simulink model "noizeGen"  (R2016b)
settings: Solver=VariableStepAuto  StartTime=0.0  StopTime=270  RelTol=1e-3
values from neighbouring files (symbols this model uses):
  noisePower = db2pow(-66)    [kalmanData.m]
  peak0amp = 0.0043080+0.0005    (= 0.004808)    [kalmanData.m]
  peak0fq = 0.003701*2*pi    (= 0.0232540688219)    [kalmanData.m]
  peak1amp = 0.0087010+0.0002    (= 0.008901)    [kalmanData.m]
  peak1fq = 0.9919*2*pi    (= 6.23229150619)    [kalmanData.m]
  peak2amp = 0.0023260+0.001    (= 0.003326)    [kalmanData.m]
  peak2fq = 2.979*2*pi    (= 18.7176090301)    [kalmanData.m]
  peak3amp = 0.0015270+0.00027    (= 0.001797)    [kalmanData.m]
  peak3fq = 4.978*2*pi    (= 31.2776964591)    [kalmanData.m]
  peak4amp = 0.0010100+0.0002    (= 0.00121)    [kalmanData.m]
  peak4fq = 6.973*2*pi    (= 43.812651147)    [kalmanData.m]
  peak5amp = 0.0009673+0.00023    (= 0.0011973)    [kalmanData.m]
  peak5fq = 8.96*2*pi    (= 56.2973403523)    [kalmanData.m]
libraries: simulink x1
settings Model: Creator=niels  LastModifiedBy=niels

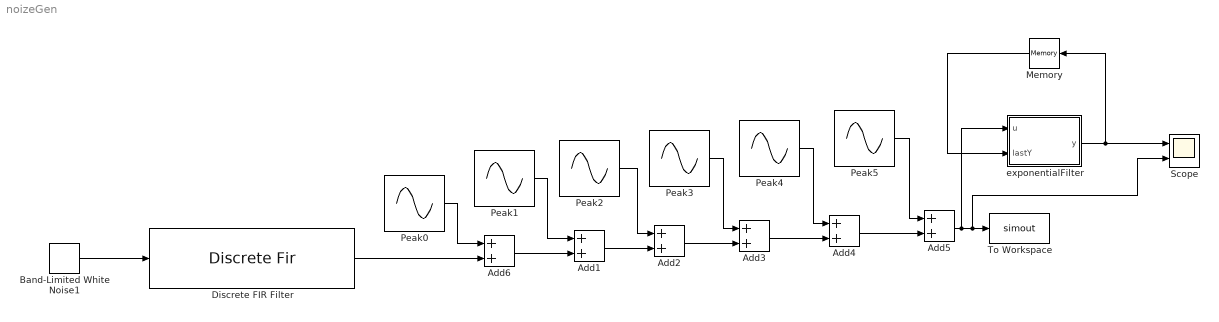
== system noizeGen ==
  Add{1..6} (6 alike) : Sum
  Band-Limited White Noise1 : simulink/Sources/Band-Limited White Noise  Cov=[noisePower]  Ts=.05  seed=[23341]
  Discrete FIR Filter : DiscreteFir  Coefficients=[1.4 2.5 0.4 0.3 0.2 0.1]
  Memory : Memory  InheritSampleTime=on
  Peak0 : Sin  Amplitude=peak0amp  Frequency=peak0fq  Phase=pi/2  SampleTime=.05
  Peak1 : Sin  Amplitude=peak1amp  Frequency=peak1fq  Phase=pi/2  SampleTime=.05
  Peak2 : Sin  Amplitude=peak2amp  Frequency=peak2fq  Phase=pi/2  SampleTime=.05
  Peak3 : Sin  Amplitude=peak3amp  Frequency=peak3fq  Phase=pi/2  SampleTime=.05
  Peak4 : Sin  Amplitude=peak4amp  Frequency=peak4fq  Phase=pi/2  SampleTime=.05
  Peak5 : Sin  Amplitude=peak5amp  Frequency=peak5fq  Phase=pi/2  SampleTime=.05
  Scope : Scope  NumInputPorts=2
  To Workspace : ToWorkspace  VariableName=simout  SaveFormat=Timeseries  SampleTime=-1
  exponentialFilter : MATLAB Function  TreatAsAtomicUnit=on  SystemSampleTime=0.05
  wires:
  Band-Limited White Noise1/1 -> Discrete FIR Filter/1
  Add1/1 -> Add2/2
  Add2/1 -> Add3/2
  Add3/1 -> Add4/2
  Add4/1 -> Add5/2
  Peak1/1 -> Add1/1
  Peak2/1 -> Add2/1
  Peak3/1 -> Add3/1
  Peak4/1 -> Add4/1
  Peak5/1 -> Add5/1
  Add5/1 -> exponentialFilter/1(u), Scope/2, To Workspace/1
  Peak0/1 -> Add6/1
  Add6/1 -> Add1/2
  Discrete FIR Filter/1 -> Add6/2
  exponentialFilter/1(y) -> Memory/1, Scope/1
  Memory/1 -> exponentialFilter/2(lastY)

== matlab function noizeGen/exponentialFilter ==
  data: u input; y output; lastY input
function y = fcn(u,lastY)

    alpha = .05;
    
    y = alpha*u + (1-alpha)* lastY;
